simulink model "model1"  (R2015b)
settings: Solver=ode3  StartTime=0.0  StopTime=4  FixedStep=0.001  RelTol=1e-3
values from neighbouring files (symbols this model uses):
  k11 = 10    [initModel1.m]
  k12 = 25    [initModel1.m]
  k21 = 10    [initModel1.m]
  k22 = 25    [initModel1.m]
  theta0 = 0.5    [initModel1.m]
  x0 = 2    [initModel1.m]
  z0 = 2.3    [initModel1.m]
undefined symbols (not defined in the file or in its folder): mod1control, pvtol
settings Model: Creator=Subodh  LastModifiedBy=Subodh
settings HardwareCC: ProdWordSize=32  ProdHWDeviceType=Specified

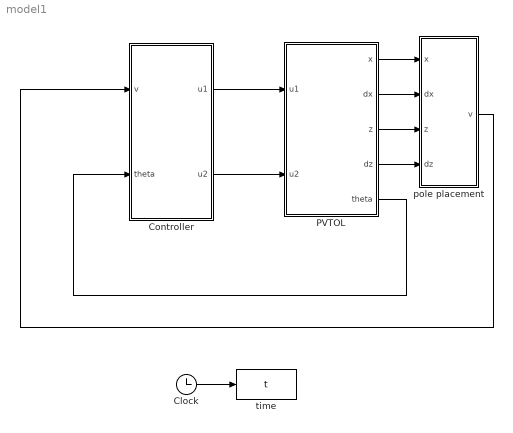
== system model1 ==
  Clock : Clock
  Controller : Subsystem
  PVTOL : Subsystem
  pole placement : Subsystem
  time : ToWorkspace  VariableName=t  SampleTime=-1
  wires:
  PVTOL/1(x) -> pole placement/1(x)
  PVTOL/2(dx) -> pole placement/2(dx)
  PVTOL/3(z) -> pole placement/3(z)
  PVTOL/4(dz) -> pole placement/4(dz)
  pole placement/1(v) -> Controller/1(v)
  PVTOL/5(theta) -> Controller/2(theta)
  Controller/1(u1) -> PVTOL/1(u1)
  Controller/2(u2) -> PVTOL/2(u2)
  Clock/1 -> time/1

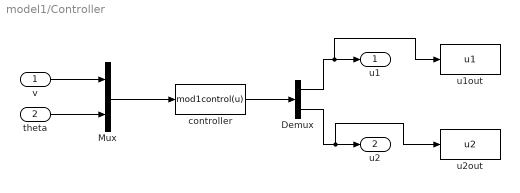
== system model1/Controller ==
  v : Inport
  theta : Inport  Port=2
  Demux : Demux  Outputs=2
  Mux : Mux  Inputs=2
  controller : MATLABFcn  MATLABFcn=mod1control(u)
  u1out : ToWorkspace  VariableName=u1  SampleTime=-1
  u2out : ToWorkspace  VariableName=u2  SampleTime=-1
  u1 : Outport
  u2 : Outport  Port=2
  wires:
  Mux/1 -> controller/1
  controller/1 -> Demux/1
  Demux/1 -> u1out/1, u1/1
  v/1 -> Mux/1
  Demux/2 -> u2out/1, u2/1
  theta/1 -> Mux/2

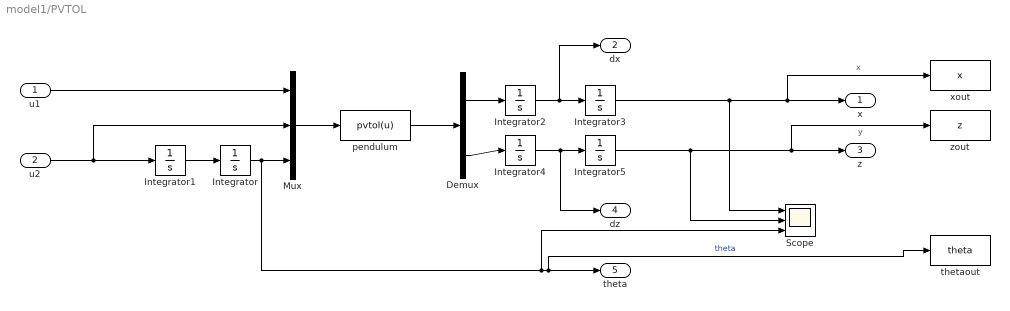
== system model1/PVTOL ==
  u1 : Inport
  u2 : Inport  Port=2
  Demux : Demux  Outputs=2
  Integrator : Integrator  InitialCondition=theta0
  Integrator1 : Integrator
  Integrator2 : Integrator
  Integrator3 : Integrator  InitialCondition=x0
  Integrator4 : Integrator
  Integrator5 : Integrator  InitialCondition=z0
  Mux : Mux  Inputs=3
  Scope : Scope  NumInputPorts=3
  pendulum : MATLABFcn  MATLABFcn=pvtol(u)  OutputDimensions=2
  thetaout : ToWorkspace  VariableName=theta  SampleTime=-1
  xout : ToWorkspace  VariableName=x  SampleTime=-1
  zout : ToWorkspace  VariableName=z  SampleTime=-1
  x : Outport
  dx : Outport  Port=2
  z : Outport  Port=3
  dz : Outport  Port=4
  theta : Outport  Port=5
  wires:
  u2/1 -> Mux/2, Integrator1/1
  Integrator3/1 -> Scope/1, xout/1, x/1  "x"
  Integrator4/1 -> dz/1, Integrator5/1
  Integrator5/1 -> Scope/2, zout/1, z/1  "y"
  Integrator2/1 -> dx/1, Integrator3/1
  Integrator/1 -> Scope/3, thetaout/1, theta/1, Mux/3  "theta"
  Demux/1 -> Integrator2/1
  Demux/2 -> Integrator4/1
  pendulum/1 -> Demux/1
  u1/1 -> Mux/1
  Integrator1/1 -> Integrator/1
  Mux/1 -> pendulum/1

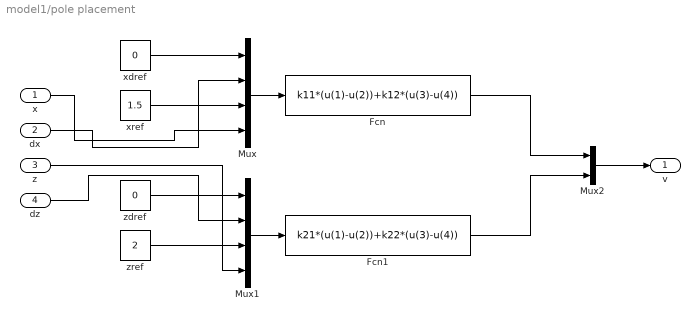
== system model1/pole placement ==
  x : Inport
  dx : Inport  Port=2
  z : Inport  Port=3
  dz : Inport  Port=4
  Fcn : Fcn  Expr=k11*(u(1)-u(2))+k12*(u(3)-u(4))
  Fcn1 : Fcn  Expr=k21*(u(1)-u(2))+k22*(u(3)-u(4))
  Mux : Mux
  Mux1 : Mux
  Mux2 : Mux  Inputs=2
  xdref : Constant  Value=0
  xref : Constant  Value=1.5
  zdref : Constant  Value=0
  zref : Constant  Value=2
  v : Outport
  wires:
  x/1 -> Mux/4
  Mux/1 -> Fcn/1
  xref/1 -> Mux/3
  zdref/1 -> Mux1/1
  dx/1 -> Mux/2
  z/1 -> Mux1/4
  dz/1 -> Mux1/2
  zref/1 -> Mux1/3
  xdref/1 -> Mux/1
  Mux1/1 -> Fcn1/1
  Fcn1/1 -> Mux2/2
  Fcn/1 -> Mux2/1
  Mux2/1 -> v/1
